simulink model "sampleModel278"  (R2021b)
settings: Solver=VariableStepAuto  StartTime=0.0  StopTime=10.0  RelTol=1e-3
undefined symbols (not defined in the file or in its folder): DiscIntNeverNeededParam, Newton, Raphson
libraries: simulink x18, slpidlib x1
settings Model: Creator=user  LastModifiedBy=user

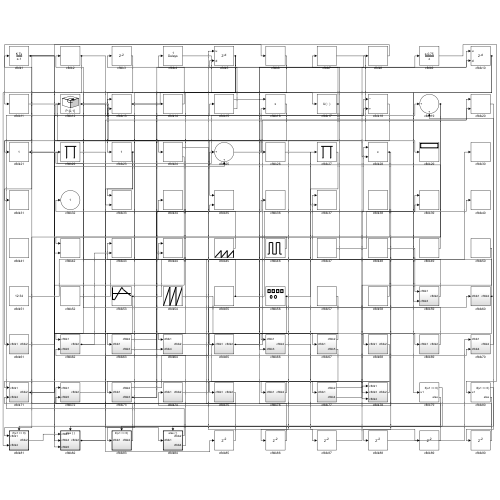
[thumbnail: Simulink's stored preview of the top-level diagram]
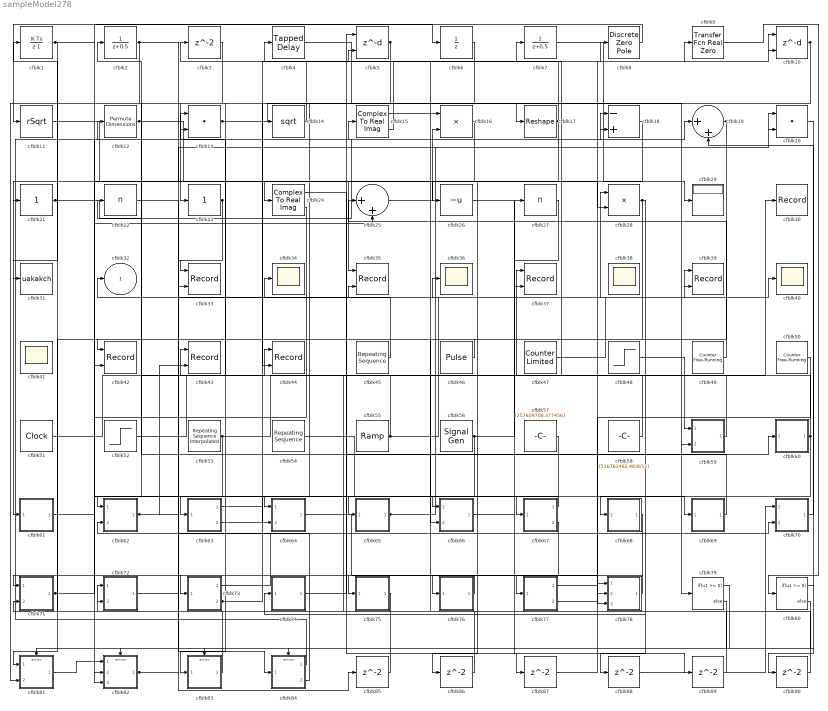
== system sampleModel278 ==
  cfblk1 : DiscreteIntegrator  ICPrevOutput=DiscIntNeverNeededParam  ICPrevScaledInput=DiscIntNeverNeededParam
  cfblk10 : Delay  DelayLengthSource=Input port  SampleTime=1
      settings: InputPortMap=u0,p1
  cfblk11 : Sqrt  Operator=rSqrt  AlgorithmType=Newton-Raphson  SaturateOnIntegerOverflow=on
  cfblk12 : PermuteDimensions
  cfblk13 : DotProduct  InputSameDT=on  OutDataTypeStr=Inherit: Inherit via internal rule
  cfblk14 : Sqrt  SaturateOnIntegerOverflow=on
  cfblk15 : ComplexToRealImag
  cfblk16 : Product  Inputs=**
  cfblk17 : Reshape
  cfblk18 : Sum  Inputs=-+
  cfblk19 : Sum  Inputs=|++
  cfblk2 : DiscreteTransferFcn  SampleTime=1
  cfblk20 : DotProduct  InputSameDT=on  OutDataTypeStr=Inherit: Inherit via internal rule
  cfblk21 : simulink/Math Operations/Slider Gain  gain=1  low=0  high=2
  cfblk22 : Product  Inputs=*
  cfblk23 : simulink/Math Operations/Slider Gain  gain=1  low=0  high=2
  cfblk24 : ComplexToRealImag
  cfblk25 : Sum  Inputs=|++
  cfblk26 : UnaryMinus
  cfblk27 : Product  Inputs=*
  cfblk28 : Product  Inputs=**
  cfblk29 : Display
  cfblk{3,85..90} (7 alike) : Delay  SampleTime=1
  cfblk30 : Record  FileSettingsInternal="{\"entries\":[{\"content\":{\"excelSettings\":{\"content\":{},\"type\":\"Streamout.ExcelSettings\"}},\"type\":\"Streamout.FileSettingStorage\",\"uuid\":\"613e592d-018a-4d70-afd0-ab2d035ef272\"}],\"packageUris\":[\"http://schema.mathworks.com/mf0/streamout_blocks/R2020a\"],\"version\":\"1.0\"}"  SignalsInternal="{\"entries\":[{\"content\":{\"signals\":[{\"content\":{\"blockPath\":[\"sampleModel278/cfblk30\"],\"channel\":[],\"dimensions\":[1],\"domain\":\"sampleModel278/cfblk30\",\"lineColor\":\"#22b573\",\"plots\":[1],\"port\":1,\"sid\":[\"\"],\"signalID\":11679,\"signalName\":\"cfblk53\"},\"type\":\"RecordBlkView.Signal\",\"uuid\":\"431496ca-f51d-4317-9847-c7ba54b4be8a\"}]},\"type\":\"RecordBlkView.InputSignals\",\"uuid\":\"2f4c0acb-aa99-4c6b-98d7-5546c209ada9\"}],\"packageUris\":[\"http://schema.mathworks.com/mf0/streamout_blocks/R2020a\"],\"version\":\"1.0\"}"  VisualizationBindings="{\"sparklinesplugin\":{\"info\":[{\"bindingParametersList\":[],\"subplotID\":1}]}}"
  cfblk31 : ToWorkspace  VariableName=uakakch  SaveFormat=Timeseries  SampleTime=-1
  cfblk33 : Record  FileSettingsInternal="{\"entries\":[{\"content\":{\"excelSettings\":{\"content\":{},\"type\":\"Streamout.ExcelSettings\"}},\"type\":\"Streamout.FileSettingStorage\",\"uuid\":\"ffadc4b8-0dfd-40c9-9b9d-69bf48ab0bda\"}],\"packageUris\":[\"http://schema.mathworks.com/mf0/streamout_blocks/R2020a\"],\"version\":\"1.0\"}"  Layout=[1 1]  SignalsInternal="{\"entries\":[{\"content\":{\"signals\":[{\"content\":{\"blockPath\":[\"sampleModel278/cfblk33\"],\"channel\":[],\"dimensions\":[1],\"domain\":\"sampleModel278/cfblk33\",\"lineColor\":\"#a2142f\",\"plots\":[1],\"port\":1,\"sid\":[\"\"],\"signalID\":11723,\"signalName\":\"cfblk23\"},\"type\":\"RecordBlkView.Signal\",\"uuid\":\"c846ee53-8b50-4807-afbd-d3711eb7dd49\"},{\"content\":{\"blockPath\":[\"sampleModel278/cfblk33\"],\"channel\":[],\"dimensions\":[1],\"domain\":\"sampleModel278/cfblk33\",\"lineColor\":\"#139fff\",\"plots\":[1],\"port\":2,\"sid\":[\"\"],\"signalID\":11727,\"signalName\":\"cfblk23\"},\"type\":\"RecordBlkView.Signal\",\"uuid\":\"cd54df4a-feda-4ff9-8210-363714cbfed4\"}]},\"type\":\"RecordBlkView.InputSignals\",\"uuid\":\"01557ded-b03f-4718-92ea-ae6b2a9ea9bd\"}],\"packageUris\":[\"http://schema.mathworks.com/mf0/streamout_blocks/R2020a\"],\"version\":\"1.0\"}"  VisualizationBindings="{\"xyplotplugin\":{\"info\":[{\"series\":[{\"bindingParametersList\":[{\"parameter\":\"X-Axis\",\"signalID\":11723,\"signalName\":\"cfblk23\"},{\"parameter\":\"Y-Axis\",\"signalID\":11727,\"signalName\":\"cfblk23\"}],\"seriesID\":14034}],\"subplotID\":1}]}}"  CompatibilityTag=XY
  cfblk{34,36,38,40..41} (5 alike) : Scope
      cfblk38 settings: Floating=on
      cfblk41 settings: Floating=on
  cfblk35 : Record  FileSettingsInternal="{\"entries\":[{\"content\":{\"excelSettings\":{\"content\":{},\"type\":\"Streamout.ExcelSettings\"}},\"type\":\"Streamout.FileSettingStorage\",\"uuid\":\"79ac4d0b-32cc-4147-9c5f-160e374bd6f1\"}],\"packageUris\":[\"http://schema.mathworks.com/mf0/streamout_blocks/R2020a\"],\"version\":\"1.0\"}"  Layout=[1 1]  SignalsInternal="{\"entries\":[{\"content\":{\"signals\":[{\"content\":{\"blockPath\":[\"sampleModel278/cfblk35\"],\"channel\":[],\"dimensions\":[1,1],\"domain\":\"sampleModel278/cfblk35\",\"lineColor\":\"#a2142f\",\"plots\":[1],\"port\":1,\"sid\":[\"\"],\"signalID\":11683,\"signalName\":\"cfblk12\"},\"type\":\"RecordBlkView.Signal\",\"uuid\":\"cee50c23-5377-4988-aab8-e70dc9d74091\"},{\"content\":{\"blockPath\":[\"sampleModel278/cfblk35\"],\"channel\":[],\"dimensions\":[1],\"domain\":\"sampleModel278/cfblk35\",\"lineColor\":\"#139fff\",\"plots\":[1],\"port\":2,\"sid\":[\"\"],\"signalID\":11687,\"signalName\":\"cfblk73:2\"},\"type\":\"RecordBlkView.Signal\",\"uuid\":\"f756d5b2-6fcb-4e95-a32a-be0f4a9c0fbb\"}]},\"type\":\"RecordBlkView.InputSignals\",\"uuid\":\"b233a160-1620-4404-bde8-9b51ab5c5cd3\"}],\"packageUris\":[\"http://schema.mathworks.com/mf0/streamout_blocks/R2020a\"],\"version\":\"1.0\"}"  VisualizationBindings="{\"xyplotplugin\":{\"info\":[{\"series\":[{\"bindingParametersList\":[{\"parameter\":\"X-Axis\",\"signalID\":11683,\"signalName\":\"cfblk12\"},{\"parameter\":\"Y-Axis\",\"signalID\":11687,\"signalName\":\"cfblk73:2\"}],\"seriesID\":45542}],\"subplotID\":1}]}}"  CompatibilityTag=XY
  cfblk37 : Record  FileSettingsInternal="{\"entries\":[{\"content\":{\"excelSettings\":{\"content\":{},\"type\":\"Streamout.ExcelSettings\"}},\"type\":\"Streamout.FileSettingStorage\",\"uuid\":\"928dffd0-792b-4854-adee-ad8a3a54d234\"}],\"packageUris\":[\"http://schema.mathworks.com/mf0/streamout_blocks/R2020a\"],\"version\":\"1.0\"}"  Layout=[1 1]  SignalsInternal="{\"entries\":[{\"content\":{\"signals\":[{\"content\":{\"blockPath\":[\"sampleModel278/cfblk37\"],\"channel\":[],\"dimensions\":[1],\"domain\":\"sampleModel278/cfblk37\",\"lineColor\":\"#a2142f\",\"plots\":[1],\"port\":1,\"sid\":[\"\"],\"signalID\":11691,\"signalName\":\"cfblk75\"},\"type\":\"RecordBlkView.Signal\",\"uuid\":\"ddc6fa25-3967-467f-baa1-9360728fba62\"},{\"content\":{\"blockPath\":[\"sampleModel278/cfblk37\"],\"channel\":[],\"dimensions\":[1],\"domain\":\"sampleModel278/cfblk37\",\"lineColor\":\"#139fff\",\"plots\":[1],\"port\":2,\"sid\":[\"\"],\"signalID\":11695,\"signalName\":\"cfblk27\"},\"type\":\"RecordBlkView.Signal\",\"uuid\":\"011298d1-e885-48b6-ac84-b8ac9bfbbe42\"}]},\"type\":\"RecordBlkView.InputSignals\",\"uuid\":\"2ccc9994-3c86-4786-a193-7a9b8578ca6a\"}],\"packageUris\":[\"http://schema.mathworks.com/mf0/streamout_blocks/R2020a\"],\"version\":\"1.0\"}"  VisualizationBindings="{\"xyplotplugin\":{\"info\":[{\"series\":[{\"bindingParametersList\":[{\"parameter\":\"X-Axis\",\"signalID\":11691,\"signalName\":\"cfblk75\"},{\"parameter\":\"Y-Axis\",\"signalID\":11695,\"signalName\":\"cfblk27\"}],\"seriesID\":6918}],\"subplotID\":1}]}}"  CompatibilityTag=XY
  cfblk39 : Record  FileSettingsInternal="{\"entries\":[{\"content\":{\"excelSettings\":{\"content\":{},\"type\":\"Streamout.ExcelSettings\"}},\"type\":\"Streamout.FileSettingStorage\",\"uuid\":\"a45da438-403e-40e9-b71e-507e939632aa\"}],\"packageUris\":[\"http://schema.mathworks.com/mf0/streamout_blocks/R2020a\"],\"version\":\"1.0\"}"  Layout=[1 1]  SignalsInternal="{\"entries\":[{\"content\":{\"signals\":[{\"content\":{\"blockPath\":[\"sampleModel278/cfblk39\"],\"channel\":[],\"dimensions\":[1],\"domain\":\"sampleModel278/cfblk39\",\"lineColor\":\"#a2142f\",\"plots\":[1],\"port\":1,\"sid\":[\"\"],\"signalID\":11731,\"signalName\":\"cfblk47\"},\"type\":\"RecordBlkView.Signal\",\"uuid\":\"eae857c1-9a3c-4252-906c-d31a20cc3c92\"},{\"content\":{\"blockPath\":[\"sampleModel278/cfblk39\"],\"channel\":[],\"dimensions\":[1],\"domain\":\"sampleModel278/cfblk39\",\"lineColor\":\"#139fff\",\"plots\":[1],\"port\":2,\"sid\":[\"\"],\"signalID\":11735,\"signalName\":\"cfblk63:2\"},\"type\":\"RecordBlkView.Signal\",\"uuid\":\"249e95c1-cc06-447c-98d2-16211a7ffd63\"}]},\"type\":\"RecordBlkView.InputSignals\",\"uuid\":\"77544bd5-671c-4e1f-a4f5-db7ee579729e\"}],\"packageUris\":[\"http://schema.mathworks.com/mf0/streamout_blocks/R2020a\"],\"version\":\"1.0\"}"  VisualizationBindings="{\"xyplotplugin\":{\"info\":[{\"series\":[{\"bindingParametersList\":[{\"parameter\":\"X-Axis\",\"signalID\":11731,\"signalName\":\"cfblk47\"},{\"parameter\":\"Y-Axis\",\"signalID\":11735,\"signalName\":\"cfblk63:2\"}],\"seriesID\":663}],\"subplotID\":1}]}}"  CompatibilityTag=XY
  cfblk4 : simulink/Discrete/Tapped Delay  vinit=0.0  samptime=-1  NumDelays=1  DelayOrder=Oldest  includeCurrent=off
  cfblk42 : Record  FileSettingsInternal="{\"entries\":[{\"content\":{\"excelSettings\":{\"content\":{},\"type\":\"Streamout.ExcelSettings\"}},\"type\":\"Streamout.FileSettingStorage\",\"uuid\":\"d6f97b6e-fb10-41bd-b103-1d8caa88e39f\"}],\"packageUris\":[\"http://schema.mathworks.com/mf0/streamout_blocks/R2020a\"],\"version\":\"1.0\"}"  Layout=[1 1]  SignalsInternal="{\"entries\":[{\"content\":{\"signals\":[{\"content\":{\"blockPath\":[\"sampleModel278/cfblk42\"],\"channel\":[],\"dimensions\":[1],\"domain\":\"sampleModel278/cfblk42\",\"lineColor\":\"#a2142f\",\"plots\":[1],\"port\":1,\"sid\":[\"\"],\"signalID\":11699,\"signalName\":\"cfblk46\"},\"type\":\"RecordBlkView.Signal\",\"uuid\":\"251f6560-360e-4ff2-ba4c-21c8b0cdd92d\"},{\"content\":{\"blockPath\":[\"sampleModel278/cfblk42\"],\"channel\":[],\"dimensions\":[1,1],\"domain\":\"sampleModel278/cfblk42\",\"lineColor\":\"#139fff\",\"plots\":[1],\"port\":2,\"sid\":[\"\"],\"signalID\":11703,\"signalName\":\"cfblk18\"},\"type\":\"RecordBlkView.Signal\",\"uuid\":\"efbb43ee-0230-4e74-b73a-26148a9d0e7b\"}]},\"type\":\"RecordBlkView.InputSignals\",\"uuid\":\"777bd1ef-2fc7-41ba-b680-345c3fc82082\"}],\"packageUris\":[\"http://schema.mathworks.com/mf0/streamout_blocks/R2020a\"],\"version\":\"1.0\"}"  VisualizationBindings="{\"xyplotplugin\":{\"info\":[{\"series\":[{\"bindingParametersList\":[{\"parameter\":\"X-Axis\",\"signalID\":11699,\"signalName\":\"cfblk46\"},{\"parameter\":\"Y-Axis\",\"signalID\":11703,\"signalName\":\"cfblk18\"}],\"seriesID\":19161}],\"subplotID\":1}]}}"  CompatibilityTag=XY
  cfblk43 : Record  FileSettingsInternal="{\"entries\":[{\"content\":{\"excelSettings\":{\"content\":{},\"type\":\"Streamout.ExcelSettings\"}},\"type\":\"Streamout.FileSettingStorage\",\"uuid\":\"49f19f1c-f43c-45ea-9add-c7aba8d2dc19\"}],\"packageUris\":[\"http://schema.mathworks.com/mf0/streamout_blocks/R2020a\"],\"version\":\"1.0\"}"  Layout=[1 1]  SignalsInternal="{\"entries\":[{\"content\":{\"signals\":[{\"content\":{\"blockPath\":[\"sampleModel278/cfblk43\"],\"channel\":[],\"dimensions\":[1],\"domain\":\"sampleModel278/cfblk43\",\"lineColor\":\"#a2142f\",\"plots\":[1],\"port\":1,\"sid\":[\"\"],\"signalID\":11707,\"signalName\":\"cfblk59\"},\"type\":\"RecordBlkView.Signal\",\"uuid\":\"f262e0a1-0dd0-4162-bc04-4042543cb925\"},{\"content\":{\"blockPath\":[\"sampleModel278/cfblk43\"],\"channel\":[],\"dimensions\":[1],\"domain\":\"sampleModel278/cfblk43\",\"lineColor\":\"#139fff\",\"plots\":[1],\"port\":2,\"sid\":[\"\"],\"signalID\":11711,\"signalName\":\"cfblk62\"},\"type\":\"RecordBlkView.Signal\",\"uuid\":\"14ac35d8-e6df-4e01-9fc3-6e9654b9195c\"}]},\"type\":\"RecordBlkView.InputSignals\",\"uuid\":\"01f5ca12-bcd0-4998-869a-9f7e36cb9a8d\"}],\"packageUris\":[\"http://schema.mathworks.com/mf0/streamout_blocks/R2020a\"],\"version\":\"1.0\"}"  VisualizationBindings="{\"xyplotplugin\":{\"info\":[{\"series\":[{\"bindingParametersList\":[{\"parameter\":\"X-Axis\",\"signalID\":11707,\"signalName\":\"cfblk59\"},{\"parameter\":\"Y-Axis\",\"signalID\":11711,\"signalName\":\"cfblk62\"}],\"seriesID\":42773}],\"subplotID\":1}]}}"  CompatibilityTag=XY
  cfblk44 : Record  FileSettingsInternal="{\"entries\":[{\"content\":{\"excelSettings\":{\"content\":{},\"type\":\"Streamout.ExcelSettings\"}},\"type\":\"Streamout.FileSettingStorage\",\"uuid\":\"f9e977a4-f4ba-4cf2-828c-4992706f1371\"}],\"packageUris\":[\"http://schema.mathworks.com/mf0/streamout_blocks/R2020a\"],\"version\":\"1.0\"}"  Layout=[1 1]  SignalsInternal="{\"entries\":[{\"content\":{\"signals\":[{\"content\":{\"blockPath\":[\"sampleModel278/cfblk44\"],\"channel\":[],\"dimensions\":[1],\"domain\":\"sampleModel278/cfblk44\",\"lineColor\":\"#a2142f\",\"plots\":[1],\"port\":1,\"sid\":[\"\"],\"signalID\":11715,\"signalName\":\"cfblk51\"},\"type\":\"RecordBlkView.Signal\",\"uuid\":\"5493c28d-61f1-4e5c-a4f0-a367b1d50efd\"},{\"content\":{\"blockPath\":[\"sampleModel278/cfblk44\"],\"channel\":[],\"dimensions\":[1],\"domain\":\"sampleModel278/cfblk44\",\"lineColor\":\"#139fff\",\"plots\":[1],\"port\":2,\"sid\":[\"\"],\"signalID\":11719,\"signalName\":\"cfblk5\"},\"type\":\"RecordBlkView.Signal\",\"uuid\":\"0b948ff4-c60d-4a33-a400-9a1c2432bf00\"}]},\"type\":\"RecordBlkView.InputSignals\",\"uuid\":\"d3a7b93b-1d37-4163-a791-6052eccdaada\"}],\"packageUris\":[\"http://schema.mathworks.com/mf0/streamout_blocks/R2020a\"],\"version\":\"1.0\"}"  VisualizationBindings="{\"xyplotplugin\":{\"info\":[{\"series\":[{\"bindingParametersList\":[{\"parameter\":\"X-Axis\",\"signalID\":11715,\"signalName\":\"cfblk51\"},{\"parameter\":\"Y-Axis\",\"signalID\":11719,\"signalName\":\"cfblk5\"}],\"seriesID\":29617}],\"subplotID\":1}]}}"  CompatibilityTag=XY
  cfblk45 : simulink/Sources/Repeating Sequence  rep_seq_t=[0 2]  rep_seq_y=[-754044833.512842, -471257157.751319]
  cfblk46 : DiscretePulseGenerator  PulseType=Time based  Amplitude=[442704016.821276]  Period=[38740735.778714]  PulseWidth=5  PhaseDelay=[4.000000]
  cfblk47 : simulink/Sources/Counter Limited  uplimit=[778.000000]  tsamp=-1
  cfblk48 : Step  Time=[44.000000]  Before=[285534383.298485]  After=[-396190397.045518]  SampleTime=0
  cfblk49 : simulink/Sources/Counter Free-Running  NumBits=[27.000000]  tsamp=-1
  cfblk5 : Delay  DelayLengthSource=Input port  SampleTime=1
      settings: InputPortMap=u0,p1
  cfblk50 : simulink/Sources/Counter Free-Running  NumBits=[54.000000]  tsamp=-1
  cfblk51 : DigitalClock
  cfblk52 : Step  Time=[21.000000]  Before=[-93639301.169280]  After=[-150879894.686397]  SampleTime=0
  cfblk53 : simulink/Sources/Repeating Sequence Interpolated  OutValues=[-820962692.471345, -952983381.611810, 916910052.502229, 574642700.696072, -338122926.781324]  TimeValues=[0 0.1 0.5 0.6 1].'  LookUpMeth=Use Input Above  tsamp=0.01  OutMin=[]  OutMax=[]  OutDataTypeStr=double  OutputDataTypeScalingMode=double  OutDataType=fixdt(0,8)  OutScaling=2^-10
  cfblk54 : simulink/Sources/Repeating Sequence  rep_seq_t=[0 2]  rep_seq_y=[378225475.621923, 919551317.298291]
  cfblk55 : simulink/Sources/Ramp  slope=[-6762.771919]  start=[19.434632]  InitialOutput=[275730.831924]
  cfblk56 : SignalGenerator  WaveForm=sawtooth  Amplitude=[-774185668.504646]  Units=rad/sec
  cfblk57 : Constant  Value=[257609708.377456]  SampleTime=1
  cfblk58 : Constant  Value=[516762482.483653]  SampleTime=1
  cfblk59 : Subsystem
  cfblk6 : UnitDelay  HasFrameUpgradeWarning=on
  cfblk60 : Subsystem
  cfblk61 : Subsystem
  cfblk62 : Subsystem
  cfblk63 : Subsystem
  cfblk64 : Subsystem
  cfblk65 : Subsystem
  cfblk66 : Subsystem
  cfblk67 : Subsystem
  cfblk68 : Subsystem
  cfblk69 : Subsystem
  cfblk7 : DiscreteTransferFcn  SampleTime=1
  cfblk70 : Subsystem
  cfblk71 : Subsystem
  cfblk72 : Subsystem
  cfblk73 : Subsystem
  cfblk74 : Subsystem
  cfblk75 : Subsystem
  cfblk76 : Subsystem
  cfblk77 : Subsystem
  cfblk78 : Subsystem
  cfblk79 : If  IfExpression=u1 >= 0  SampleTime=1
  cfblk8 : DiscreteZeroPole  Poles=[0 0.5]  Gain=1
  cfblk80 : If  IfExpression=u1 >= 0  SampleTime=1
  cfblk81 : Subsystem  TreatAsAtomicUnit=on
  cfblk82 : Subsystem  TreatAsAtomicUnit=on
  cfblk83 : Subsystem  TreatAsAtomicUnit=on
  cfblk84 : Subsystem  TreatAsAtomicUnit=on
  cfblk9 : simulink/Discrete/Transfer Fcn Real Zero  ZeroZ=0.75  ICPrevInput=0.0  DoSatur=off
      settings: SourceProductBaseCode=SL
  cfblk32 : Outport
  wires:
  cfblk11/1 -> cfblk24/1
  cfblk46/1 -> cfblk42/1
  cfblk3/1 -> cfblk23/1
  cfblk21/1 -> cfblk19/1, cfblk69/1(cfblk1)
  cfblk68/1(cfblk2) -> cfblk75/1(cfblk1)
  cfblk8/1 -> cfblk11/1
  cfblk75/1(cfblk2) -> cfblk37/1
  cfblk7/1 -> cfblk29/1
  cfblk27/1 -> cfblk37/2
  cfblk28/1 -> cfblk74/1(cfblk1), cfblk81/1(cfblk1)
  cfblk12/1 -> cfblk35/1, cfblk18/2
  cfblk84/1(cfblk2) -> cfblk12/1
  cfblk16/1 -> cfblk61/1(cfblk1)
  cfblk60/1(cfblk2) -> cfblk68/1(cfblk1), cfblk13/2
  cfblk22/1 -> cfblk84/1(cfblk1)
  cfblk83/1(cfblk2) -> cfblk72/1(cfblk1)
  cfblk6/1 -> cfblk64/1(cfblk1)
  cfblk59/1(cfblk2) -> cfblk43/1
  cfblk81/1(cfblk2) -> cfblk82/1(cfblk1)
  cfblk56/1 -> cfblk27/1, cfblk65/1(cfblk1)
  cfblk51/1 -> cfblk44/1
  cfblk69/1(cfblk2) -> cfblk22/1
  cfblk13/1 -> cfblk17/1, cfblk8/1
  cfblk25/1 -> cfblk16/2
  cfblk70/1(cfblk2) -> cfblk19/2
  cfblk78/1(cfblk2) -> cfblk71/1(cfblk1)
  cfblk17/1 -> cfblk4/1, cfblk86/1
  cfblk19/1 -> cfblk66/2(cfblk3), cfblk88/1
  cfblk65/1(cfblk2) -> cfblk20/1, cfblk10/2
  cfblk67/1(cfblk2) -> cfblk66/1(cfblk1)
  cfblk14/1 -> cfblk3/1
  cfblk5/1 -> cfblk62/1(cfblk1), cfblk83/1(cfblk1), cfblk44/2
  cfblk77/1(cfblk2) -> cfblk40/1
  cfblk53/1 -> cfblk82/2(cfblk4), cfblk30/1
  cfblk71/1(cfblk2) -> cfblk13/1, cfblk25/2
  cfblk45/1 -> cfblk32/1
  cfblk57/1 -> cfblk63/1(cfblk1)
  cfblk47/1 -> cfblk39/1
  cfblk50/1 -> cfblk78/2(cfblk3)
  cfblk62/1(cfblk2) -> cfblk20/2, cfblk43/2
  cfblk55/1 -> cfblk28/1, cfblk2/1
  cfblk1/1 -> cfblk31/1, cfblk6/1, cfblk26/1, cfblk64/2(cfblk4)
  cfblk63/1(cfblk2) -> cfblk36/1
  cfblk2/1 -> cfblk28/2, cfblk21/1
  cfblk58/1 -> cfblk7/1
  cfblk73/1(cfblk2) -> cfblk5/1
  cfblk15/1 -> cfblk9/1
  cfblk61/1(cfblk2) -> cfblk15/1
  cfblk73/2(cfblk3) -> cfblk35/2, cfblk18/1
  cfblk23/1 -> cfblk33/1, cfblk33/2
  cfblk4/1 -> cfblk79/1
  cfblk67/2(cfblk5) -> cfblk76/1(cfblk1)
  cfblk24/2 -> cfblk82/3(cfblk5)
  cfblk84/2(cfblk4) -> cfblk62/2(cfblk5)
  cfblk18/1 -> cfblk42/2
  cfblk48/1 -> cfblk59/1(cfblk1)
  cfblk54/1 -> cfblk67/1(cfblk1)
  cfblk77/2(cfblk4) -> cfblk10/1
  cfblk74/1(cfblk2) -> cfblk60/1(cfblk1)
  cfblk82/1(cfblk2) -> cfblk34/1, cfblk85/1
  cfblk63/2(cfblk3) -> cfblk39/2
  cfblk15/2 -> cfblk5/2
  cfblk26/1 -> cfblk78/3(cfblk4)
  cfblk10/1 -> cfblk59/2(cfblk3), cfblk81/2(cfblk4)
  cfblk52/1 -> cfblk14/1
  cfblk76/1(cfblk2) -> cfblk73/1(cfblk1)
  cfblk49/1 -> cfblk25/1
  cfblk9/1 -> cfblk80/1
  cfblk64/1(cfblk2) -> cfblk77/1(cfblk1)
  cfblk72/1(cfblk2) -> cfblk70/2(cfblk4)
  cfblk79/1 -> cfblk81/Action
  cfblk79/2 -> cfblk82/Action
  cfblk80/1 -> cfblk83/Action
  cfblk80/2 -> cfblk84/Action
  cfblk85/1 -> cfblk1/1
  cfblk86/1 -> cfblk71/2(cfblk4)
  cfblk24/1 -> cfblk87/1
  cfblk87/1 -> cfblk78/1(cfblk1)
  cfblk88/1 -> cfblk70/1(cfblk1)
  cfblk66/1(cfblk2) -> cfblk89/1
  cfblk89/1 -> cfblk72/2(cfblk5)
  cfblk20/1 -> cfblk90/1
  cfblk90/1 -> cfblk16/1

== system sampleModel278/cfblk59 ==
  cfblk1 : Inport
  cfblk3 : Inport  Port=2
  cfblk2 : Outport
  wires:
  cfblk3/1 -> cfblk2/1

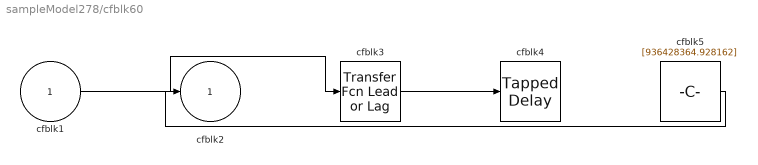
== system sampleModel278/cfblk60 ==
  cfblk1 : Inport
  cfblk3 : simulink/Discrete/Transfer Fcn Lead or Lag  PoleZ=0.95  ZeroZ=0.75  ICPrevOutput=0.0  ICPrevInput=0.0  DoSatur=off
      settings: SourceProductBaseCode=SL
  cfblk4 : simulink/Discrete/Tapped Delay  vinit=0.0  samptime=-1  NumDelays=1  DelayOrder=Oldest  includeCurrent=off
  cfblk5 : Constant  Value=[936428364.928162]  SampleTime=1
  cfblk2 : Outport
  wires:
  cfblk1/1 -> cfblk3/1
  cfblk3/1 -> cfblk4/1
  cfblk5/1 -> cfblk2/1

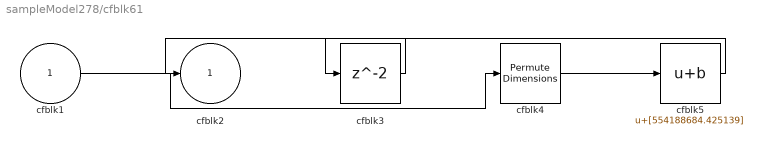
== system sampleModel278/cfblk61 ==
  cfblk1 : Inport
  cfblk3 : Delay  SampleTime=1
  cfblk4 : PermuteDimensions
  cfblk5 : Bias  Bias=[554188684.425139]
  cfblk2 : Outport
  wires:
  cfblk5/1 -> cfblk3/1
  cfblk4/1 -> cfblk5/1
  cfblk1/1 -> cfblk4/1
  cfblk3/1 -> cfblk2/1

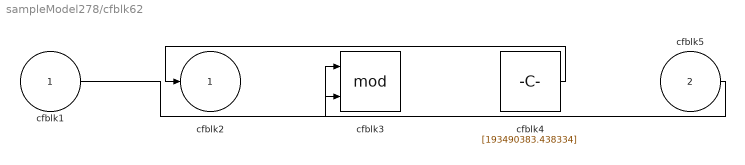
== system sampleModel278/cfblk62 ==
  cfblk1 : Inport
  cfblk5 : Inport  Port=2
  cfblk3 : Math  Operator=mod  SaturateOnIntegerOverflow=on
  cfblk4 : Constant  Value=[193490383.438334]  SampleTime=1
  cfblk2 : Outport
  wires:
  cfblk4/1 -> cfblk2/1
  cfblk5/1 -> cfblk3/1
  cfblk1/1 -> cfblk3/2

== system sampleModel278/cfblk63 ==
  cfblk1 : Inport
  cfblk2 : Outport
  cfblk3 : Outport  Port=2
  wires:
  cfblk1/1 -> cfblk2/1, cfblk3/1

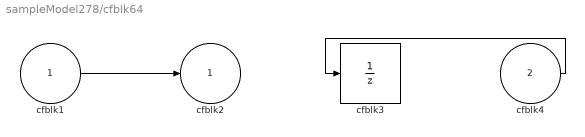
== system sampleModel278/cfblk64 ==
  cfblk1 : Inport
  cfblk4 : Inport  Port=2
  cfblk3 : UnitDelay  HasFrameUpgradeWarning=on
  cfblk2 : Outport
  wires:
  cfblk4/1 -> cfblk3/1
  cfblk1/1 -> cfblk2/1

== system sampleModel278/cfblk65 ==
  cfblk1 : Inport
  cfblk3 : slpidlib/PID Controller  Controller=PID  Form=Parallel  TimeDomain=Discrete-time  UseExternalTs=off  SampleTime=1  IntegratorMethod=Forward Euler  FilterMethod=Forward Euler  ControllerParametersSource=internal  P=1  I=1  D=0  UseFilter=on  N=100  TunerSelectOption=Transfer Function Based (PID Tuner App)  InitialConditionSource=internal  InitialConditionForIntegrator=0  InitialConditionForFilter=0  DifferentiatorICPrevScaledInput=0  ExternalReset=none  TrackingMode=off  Kt=1  LimitOutput=off  SatLimitsSource=internal  UpperSaturationLimit=inf  LowerSaturationLimit=-inf  LinearizeAsGain=off  AntiWindupMode=none  Kb=1  POutMin=[]  POutMax=[]  IOutMin=[]  IOutMax=[]  DOutMin=[]  DOutMax=[]  NOutMin=[]  NOutMax=[]  SumOutMin=[]  SumOutMax=[]  SaturationOutMin=[]  SaturationOutMax=[]  PParamMin=[]  PParamMax=[]  IParamMin=[]  IParamMax=[]  DParamMin=[]  DParamMax=[]  NParamMin=[]  NParamMax=[]  KbParamMin=[]  KbParamMax=[]  KtParamMin=[]  KtParamMax=[]  KbOutMin=[]  KbOutMax=[]  KtOutMin=[]  KtOutMax=[]  IntegratorOutMin=[]  IntegratorOutMax=[]  FilterOutMin=[]  FilterOutMax=[]  SumI1OutMin=[]  SumI1OutMax=[]  SumI2OutMin=[]  SumI2OutMax=[]  SumI3OutMin=[]  SumI3OutMax=[]  SumI4OutMin=[]  SumI4OutMax=[]  SumDOutMin=[]  SumDOutMax=[]  DifferentiatorOutMin=[]  DifferentiatorOutMax=[]  FilterDiffOutCoefMin=[]  FilterDiffOutCoefMax=[]  ReciprocalOutMin=[]  ReciprocalOutMax=[]  SumDenOutMin=[]  SumDenOutMax=[]  SumNumOutMin=[]  SumNumOutMax=[]  DivideOutMin=[]  DivideOutMax=[]  UdiffTsProdOutMin=[]  UdiffTsProdOutMax=[]  NTsProdOutMin=[]  NTsProdOutMax=[]  UintegralTsProdOutMin=[]  UintegralTsProdOutMax=[]  UngainTsProdOutMin=[]  UngainTsProdOutMax=[]  IntegratorContinuousStateAttributes=''  IntegratorStateMustResolveToSignalObject=off  IntegratorRTWStateStorageClass=Auto  FilterContinuousStateAttributes=''  FilterStateMustResolveToSignalObject=off  FilterRTWStateStorageClass=Auto  ParallelPVariant=InternalParameters  IdealPVariant=Disabled  IVariant=InternalParameters  DVariant=InternalParameters  IntegratorVariant=Discrete  SatVariant=Disabled  AWVariant=Passthrough  PCopyVariant=Disabled  TRVariant=Disabled  FdbkBlocksVariant=Forward  IdealPFdbkVariant=Disabled  SatFdbkVariant=Disabled  DerivativeFilterVariant=ForwardEulerFilter  NVariant=InternalParameters  NCopyVariant=Disabled  FilterICVariant=InternalICsFilter  IntegratorICVariant=InternalICs  ExternalResetVariant=Disabled  TRSumVariant=Passthrough  SumFdbkVariant=Disabled  SumVariant=Sum_PID  TsampFilterVariant=InternalTs  TsampNgainVariant=Passthrough  TsampIntegralVariant=Passthrough  ExternalSaturationOutDataTypeStr=Inherit: Same as second input
  cfblk2 : Outport
  wires:
  cfblk1/1 -> cfblk3/1
  cfblk3/1 -> cfblk2/1

== system sampleModel278/cfblk66 ==
  cfblk1 : Inport
  cfblk3 : Inport  Port=2
  cfblk2 : Outport
  wires:
  cfblk1/1 -> cfblk2/1

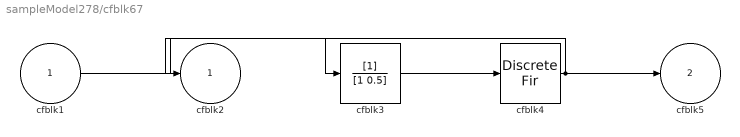
== system sampleModel278/cfblk67 ==
  cfblk1 : Inport
  cfblk3 : DiscreteFilter  SampleTime=1
  cfblk4 : DiscreteFir  SampleTime=1
  cfblk2 : Outport
  cfblk5 : Outport  Port=2
  wires:
  cfblk4/1 -> cfblk5/1, cfblk2/1
  cfblk1/1 -> cfblk3/1
  cfblk3/1 -> cfblk4/1

== system sampleModel278/cfblk68 ==
  cfblk1 : Inport
  cfblk3 : Delay  DelayLengthSource=Input port  SampleTime=1
      settings: InputPortMap=u0,p1
  cfblk4 : Constant  Value=[-50827859.087769]  SampleTime=1
  cfblk2 : Outport
  wires:
  cfblk4/1 -> cfblk2/1
  cfblk1/1 -> cfblk3/1, cfblk3/2

== system sampleModel278/cfblk69 ==
  cfblk1 : Inport
  cfblk3 : Bias  Bias=[-483781049.236620]
  cfblk4 : simulink/Math Operations/MinMax Running Resettable  Function=min  vinit=0.0
  cfblk2 : Outport
  wires:
  cfblk3/1 -> cfblk2/1
  cfblk1/1 -> cfblk4/1, cfblk4/2
  cfblk4/1 -> cfblk3/1

== system sampleModel278/cfblk70 ==
  cfblk1 : Inport
  cfblk4 : Inport  Port=2
  cfblk3 : Sin  TimeSource=Use external signal  SampleTime=0
  cfblk2 : Outport
  wires:
  cfblk1/1 -> cfblk3/1
  cfblk3/1 -> cfblk2/1

== system sampleModel278/cfblk71 ==
  cfblk1 : Inport
  cfblk4 : Inport  Port=2
  cfblk3 : simulink/Discrete/Transfer Fcn First Order  PoleZ=0.95  ICPrevOutput=0.0  DoSatur=off
  cfblk2 : Outport
  wires:
  cfblk4/1 -> cfblk2/1
  cfblk1/1 -> cfblk3/1

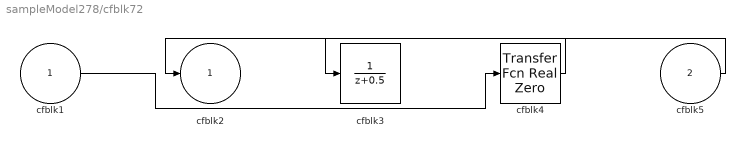
== system sampleModel278/cfblk72 ==
  cfblk1 : Inport
  cfblk5 : Inport  Port=2
  cfblk3 : DiscreteTransferFcn  SampleTime=1
  cfblk4 : simulink/Discrete/Transfer Fcn Real Zero  ZeroZ=0.75  ICPrevInput=0.0  DoSatur=off
      settings: SourceProductBaseCode=SL
  cfblk2 : Outport
  wires:
  cfblk5/1 -> cfblk2/1
  cfblk1/1 -> cfblk4/1
  cfblk4/1 -> cfblk3/1

== system sampleModel278/cfblk73 ==
  cfblk1 : Inport
  cfblk2 : Outport
  cfblk3 : Outport  Port=2
  wires:
  cfblk1/1 -> cfblk3/1, cfblk2/1

== system sampleModel278/cfblk74 ==
  cfblk1 : Inport
  cfblk3 : Product
  cfblk2 : Outport
  wires:
  cfblk1/1 -> cfblk3/1, cfblk3/2
  cfblk3/1 -> cfblk2/1

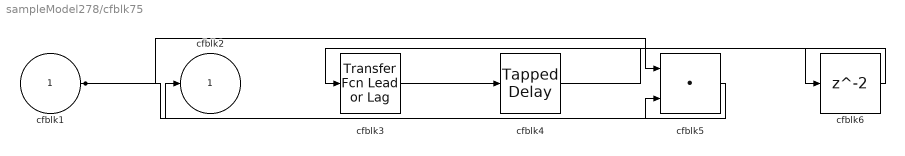
== system sampleModel278/cfblk75 ==
  cfblk1 : Inport
  cfblk3 : simulink/Discrete/Transfer Fcn Lead or Lag  PoleZ=0.95  ZeroZ=0.75  ICPrevOutput=0.0  ICPrevInput=0.0  DoSatur=off
      settings: SourceProductBaseCode=SL
  cfblk4 : simulink/Discrete/Tapped Delay  vinit=0.0  samptime=-1  NumDelays=1  DelayOrder=Oldest  includeCurrent=off
  cfblk5 : DotProduct  InputSameDT=on  OutDataTypeStr=Inherit: Inherit via internal rule
  cfblk6 : Delay  SampleTime=1
  cfblk2 : Outport
  wires:
  cfblk5/1 -> cfblk2/1
  cfblk3/1 -> cfblk4/1
  cfblk1/1 -> cfblk5/1, cfblk5/2
  cfblk4/1 -> cfblk6/1
  cfblk6/1 -> cfblk3/1

== system sampleModel278/cfblk76 ==
  cfblk1 : Inport
  cfblk3 : DiscreteIntegrator  ICPrevOutput=DiscIntNeverNeededParam  ICPrevScaledInput=DiscIntNeverNeededParam
  cfblk4 : UnaryMinus
  cfblk2 : Outport
  wires:
  cfblk4/1 -> cfblk3/1
  cfblk1/1 -> cfblk4/1
  cfblk3/1 -> cfblk2/1

== system sampleModel278/cfblk77 ==
  cfblk1 : Inport
  cfblk3 : Reshape
  cfblk2 : Outport
  cfblk4 : Outport  Port=2
  wires:
  cfblk1/1 -> cfblk3/1
  cfblk3/1 -> cfblk4/1, cfblk2/1

== system sampleModel278/cfblk78 ==
  cfblk1 : Inport
  cfblk3 : Inport  Port=2
  cfblk4 : Inport  Port=3
  cfblk2 : Outport
  wires:
  cfblk3/1 -> cfblk2/1

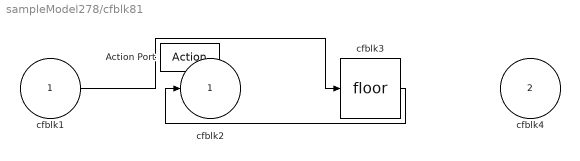
== system sampleModel278/cfblk81 ==
  cfblk1 : Inport
  cfblk4 : Inport  Port=2
  Action Port : ActionPort  ActionPortLabel=if(u1 >= 0)
  cfblk3 : Rounding
  cfblk2 : Outport
  wires:
  cfblk3/1 -> cfblk2/1
  cfblk1/1 -> cfblk3/1

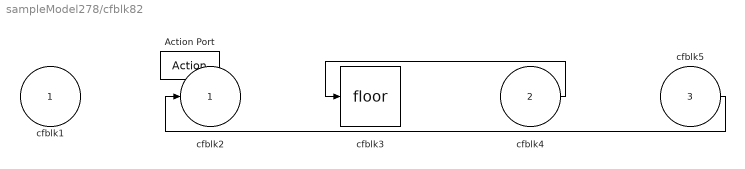
== system sampleModel278/cfblk82 ==
  cfblk1 : Inport
  cfblk4 : Inport  Port=2
  cfblk5 : Inport  Port=3
  Action Port : ActionPort  ActionPortLabel=else
  cfblk3 : Rounding
  cfblk2 : Outport
  wires:
  cfblk4/1 -> cfblk3/1
  cfblk5/1 -> cfblk2/1

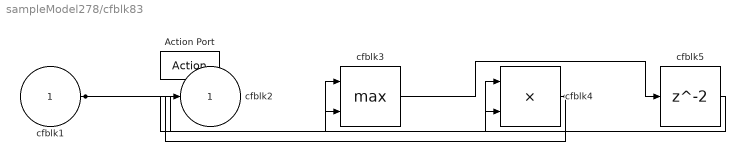
== system sampleModel278/cfblk83 ==
  cfblk1 : Inport
  Action Port : ActionPort  ActionPortLabel=if(u1 >= 0)
  cfblk3 : MinMax  Function=max  Inputs=2
  cfblk4 : Product  Inputs=**
  cfblk5 : Delay
  cfblk2 : Outport
  wires:
  cfblk1/1 -> cfblk4/1, cfblk3/1
  cfblk4/1 -> cfblk2/1, cfblk3/2
  cfblk3/1 -> cfblk5/1
  cfblk5/1 -> cfblk4/2

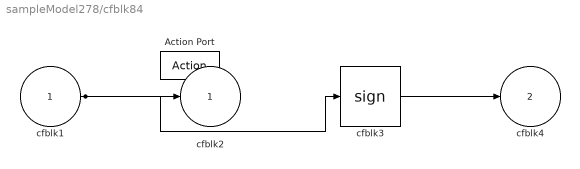
== system sampleModel278/cfblk84 ==
  cfblk1 : Inport
  Action Port : ActionPort  ActionPortLabel=else
  cfblk3 : Signum
  cfblk2 : Outport
  cfblk4 : Outport  Port=2
  wires:
  cfblk3/1 -> cfblk4/1
  cfblk1/1 -> cfblk2/1, cfblk3/1
